simulink model "threephasevsi_v1_1"  (R2021a)
settings: Solver=VariableStepAuto  StartTime=0.0  StopTime=10.0  RelTol=1e-3
settings Model: Creator=danesh  LastModifiedBy=danesh

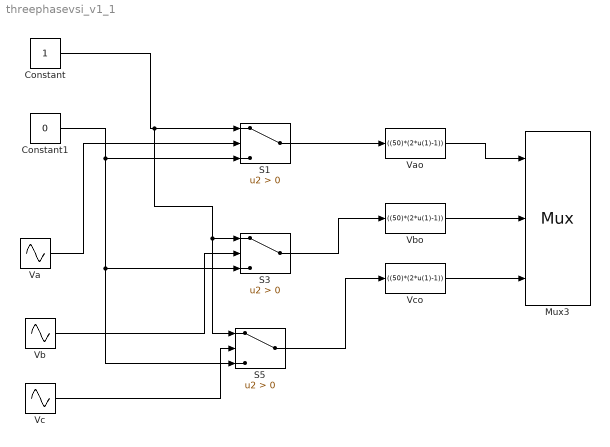
== system threephasevsi_v1_1 ==
  Constant : Constant
  Constant1 : Constant  Value=0
  Mux3 : Mux  Inputs=3
  S1 : Switch  Criteria=u2 > Threshold
  S3 : Switch  Criteria=u2 > Threshold
  S5 : Switch  Criteria=u2 > Threshold
  Va : Sin  Frequency=2*pi*50  SampleTime=0
  Vao : Fcn  Expr=((50)*(2*u(1)-1))
  Vb : Sin  Frequency=2*pi*50  Phase=-2.0904  SampleTime=0
  Vbo : Fcn  Expr=((50)*(2*u(1)-1))
  Vc : Sin  Frequency=2*pi*50  Phase=-4.188  SampleTime=0
  Vco : Fcn  Expr=((50)*(2*u(1)-1))
  wires:
  Va/1 -> S1/2
  Vco/1 -> Mux3/3
  Vbo/1 -> Mux3/2
  S3/1 -> Vbo/1
  Constant/1 -> S3/1, S5/1, S1/1
  Vb/1 -> S3/2
  S5/1 -> Vco/1
  Vc/1 -> S5/2
  S1/1 -> Vao/1
  Constant1/1 -> S1/3, S3/3, S5/3
  Vao/1 -> Mux3/1
